simulink model "Question2_v2"  (R2018a)
settings: Solver=FixedStepAuto  StartTime=0.0  StopTime=20  FixedStep=0.01  RelTol=1e-3
undefined symbols (not defined in the file): mu1, mu2, y1, y2
settings Model: Creator=Ersin Keskin  LastModifiedBy=Ersin Keskin

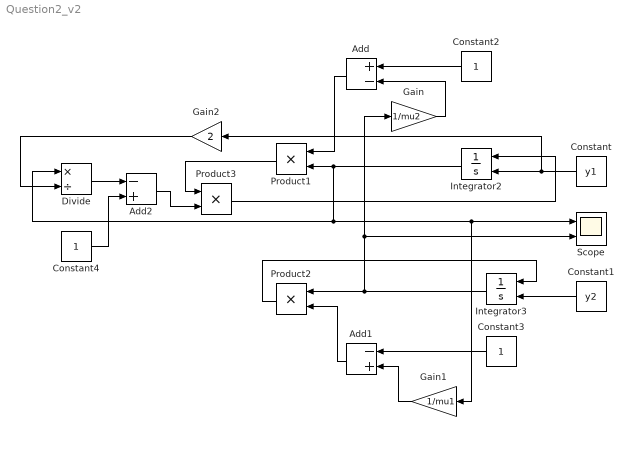
== system Question2_v2 ==
  Add : Sum  Inputs=+-
  Add1 : Sum  Inputs=-+
  Add2 : Sum  Inputs=-+
  Constant : Constant  Value=y1
  Constant1 : Constant  Value=y2
  Constant2 : Constant
  Constant3 : Constant
  Constant4 : Constant
  Divide : Product  Inputs=*/
  Gain : Gain  Gain=1/mu2
  Gain1 : Gain  Gain=1/mu1
  Gain2 : Gain  Gain=2
  Integrator2 : Integrator  InitialConditionSource=external
  Integrator3 : Integrator  InitialConditionSource=external
  Product1 : Product
  Product2 : Product
  Product3 : Product
  Scope : Scope  NumInputPorts=2
  wires:
  Product2/1 -> Integrator3/1
  Constant2/1 -> Add/1
  Gain/1 -> Add/2
  Integrator2/1 -> Gain1/1, Scope/1, Divide/1, Product1/2
  Add/1 -> Product1/1
  Constant/1 -> Gain2/1, Integrator2/2
  Integrator3/1 -> Gain/1, Scope/2, Product2/1
  Constant1/1 -> Integrator3/2
  Constant3/1 -> Add1/1
  Add1/1 -> Product2/2
  Gain1/1 -> Add1/2
  Gain2/1 -> Divide/2
  Divide/1 -> Add2/1
  Constant4/1 -> Add2/2
  Product3/1 -> Integrator2/1
  Add2/1 -> Product3/2
  Product1/1 -> Product3/1
